simulink model "MotorTestHarness"  (R2024b)
settings: Solver=VariableStepAuto  StartTime=0.0  StopTime=300  RelTol=1e-3  AbsTol=1e-3
libraries: fl_lib x12, nesl_utility x6, simulink x2
settings Model: Creator=saprasad  LastModifiedBy=jjha
settings SolverCC: AutoScaleAbsTol=off  AlgebraicLoopSolver=TrustRegion  MaxZcPerStep=1
settings DebuggingCC: UnconnectedInputMsg=warning  UnconnectedOutputMsg=warning  UnconnectedLineMsg=warning  SymbolicDimsDataTypeCodeGenerationDiagnostic=none
settings ModelReferenceCC: EnableRefExpFcnMdlSchedulingChecks=on
settings SFSimCC: CustomCodeUndefinedFunction=UseInterfaceOnly
settings RTWCC: GPUComputeCapability=3.5  DLArmComputeVersion=19.05
settings SimscapeCC: SimscapeLogType=all  SimscapeLogSimulationStatistics=on  SimscapeLogDataHistory=10000

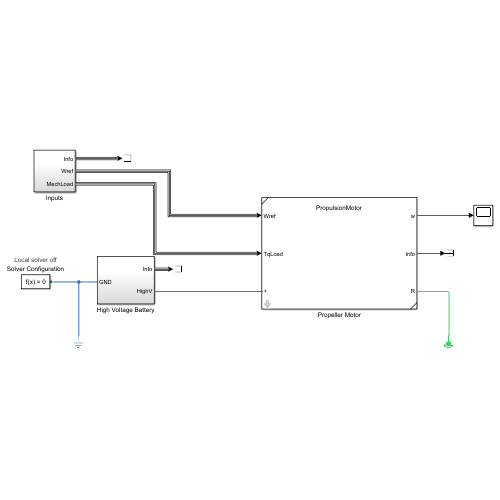
[thumbnail: Simulink's stored preview of the top-level diagram]
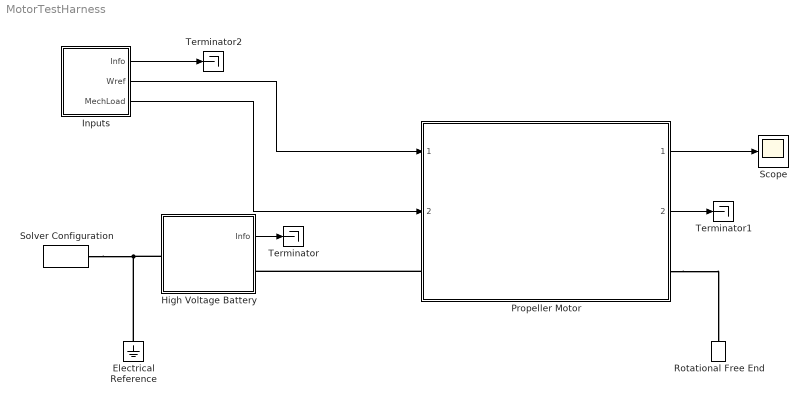
== system MotorTestHarness ==
  Electrical Reference : fl_lib/Electrical/Electrical Elements/Electrical Reference
  High Voltage Battery : Subsystem
  Inputs : Subsystem
  Propeller Motor : Subsystem  ReferencedSubsystem=PropulsionMotor  Kp=0.0129  Ki=0.00568  Kd=0.00644  N=382
  Rotational Free End : fl_lib/Mechanical/Rotational Elements/Rotational Free End  w_specify=off  w_priority=None  w=0 rad/s  w_nominal_specify=off  w_nominal_value=1  w_nominal_unit=rad/s
  Scope : Scope
  Solver Configuration : nesl_utility/Solver Configuration  PhysicalDomain=network_engine_domain  SubClassName=solver  LeftPortType=input  RightPortType=generic  Tones=[]  Harmonics=[]  SimulateNoise=off  Profile=off  UseLocalSampling=off  EnableSwitchedLinearOptims=on  FrequencyDomain=off  UseCCode=off  RelTol=0.001  AbsTol=1e-06  MinStep=1e-09  ToWorkspace=off  RevertToSquareIcSolve=off  NumHomotopyIterations=100  PhasorMode=off  PhasorModeNumHarmonics=1  ConsistencySolver=NEWTON_XTOL_AFTER_FTOL  IndexReductionMethod=DerivativeReplacement  DoDC=off  ResidualTolerance=1e-09  ConsistencyTolSource=GLOBAL  ConsistencyAbsTol=0.001  ConsistencyRelTol=0.001  ConsistencyTolFactor=0.001  UseLocalSolver=off  LocalSolverChoice=NE_BACKWARD_EULER_ADVANCER  ResolveIndetEquations=on  FunctionEvalNumThread=1  LocalSolverSampleTime=0.001  DoFixedCost=off  MaxNonlinIter=3  MaxModeIter=2  ComputeImpulses=off  ImpulseIterations=2  LinearAlgebra=auto  LinearAlgebraNumThread=0  EquationFormulation=NE_TIME_EF  DelaysMemoryBudget=1024  AutomaticFiltering=on  FilteringTimeConstant=0.001  PartitionStorageMethod=AS_NEEDED  PartitionMemoryBudget=1024  PartitionMethod=ROBUST  MultibodyUseLocalSolver=off  MultibodyLocalSolverChoice=ODE1  MultibodyLocalSolverSampleTime=0.001
      settings: AttributesFormatString=Local solver %<UseLocalSolver>
  Terminator : Terminator
  Terminator1 : Terminator
  Terminator2 : Terminator
  wires:
  Inputs/2(Wref) -> Propeller Motor/1
  Inputs/1(Info) -> Terminator2/1
  Inputs/3(MechLoad) -> Propeller Motor/2
  High Voltage Battery/1(Info) -> Terminator/1
  Propeller Motor/1 -> Scope/1
  Propeller Motor/2 -> Terminator1/1
  connections:
  High Voltage Battery/LConn1 -- Electrical Reference/LConn1 -- Solver Configuration/RConn1
  Propeller Motor/LConn1 -- High Voltage Battery/RConn1
  Propeller Motor/RConn1 -- Rotational Free End/LConn1

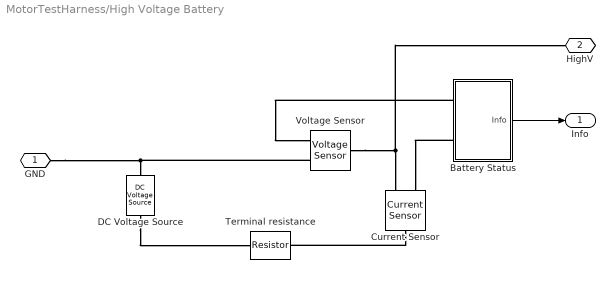
== system MotorTestHarness/High Voltage Battery ==
  Battery Status : Subsystem
  Current Sensor : fl_lib/Electrical/Electrical Sensors/Current Sensor
  DC Voltage Source : fl_lib/Electrical/Electrical Sources/DC Voltage Source  v0=420 V
      settings: AttributesFormatString=%<v0> [%<v0_unit>]
  Terminal resistance : fl_lib/Electrical/Electrical Elements/Resistor  R=0.01 Ohm  i_specify=off  i_priority=High  i=0 A  i_nominal_specify=off  i_nominal_value=1  i_nominal_unit=A  v_specify=off  v_priority=High  v=0 V  v_nominal_specify=off  v_nominal_value=1  v_nominal_unit=V
      settings: AttributesFormatString=%<R> [%<R_unit>]
  Voltage Sensor : fl_lib/Electrical/Electrical Sensors/Voltage Sensor
  GND : PMIOPort  Side=Left
  HighV : PMIOPort  Port=2  Side=Right
  Info : Outport
  wires:
  Battery Status/1(Info) -> Info/1
  connections:
  DC Voltage Source/RConn1 -- GND/RConn1 -- Voltage Sensor/RConn2
  Battery Status/LConn2 -- Current Sensor/RConn1
  Voltage Sensor/LConn1 -- HighV/RConn1 -- Current Sensor/RConn2
  Current Sensor/LConn1 -- Terminal resistance/RConn1
  DC Voltage Source/LConn1 -- Terminal resistance/LConn1
  Battery Status/LConn1 -- Voltage Sensor/RConn1

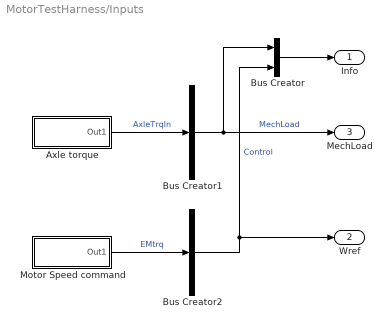
== system MotorTestHarness/Inputs ==
  Axle torque : Subsystem  mask(Continuous Multi-Step Signal){dataPoints=[0 20 0.1;60 100 0.25;105 200 0.15;205 300 0], deltaT=0.1}
      mask prompts: dataPoints "Data points"; deltaT "Interpolation step [s]"
      mask help:
      | This block generates a signal consisting of smoothly connected flat segments. Data points parameter takes an N-by-3 matrix where each row specifies a flat segment. First column and second column define start and end time of the segment, respectively. Third column defines the value of the segment. Second column can also be NaN to define a point value. Flat segments and point values are smoothly interpolated by Akima spline with the specified interpolation step.
      |
      | For example, a matrix [0 1 5; 3 nan 9; 6 8 7] for Data points defines a signal as follows. First row defines a flat segment from t=0 to t=1 of value 5. Second row defines a point at t=3 of value 9. Third row defines a flat segment from t=6 to t=8 of value 7.
      mask init:
      | sig = SignalDesigner("ContinuousMultiStep");
      | 
      | % Initialization function can access parameter names directly
      | sig.XYData = dataPoints;
      | sig.DeltaX = deltaT;
      | 
      | update(sig)
      | 
      | SignalSourceBlockCallback.setDataToLookupTableBlock( ...
      |   SignalObject = sig, ...
      |   PathToBlock = [gcb '/1-D Lookup Table']);
      mask DialogControl Control3 Prompt: horizontal spacer 1
      mask DialogControl Control4 Prompt: horizontal spacer 2
      mask DialogControl Control5 Prompt: horizontal spacer 3
      mask DialogControl PlotButton Prompt: Plot
      mask DialogControl PlotButton Callback: SignalSourceBlockCallback.plotContinuousMultiStep(gcb);
      mask Display: disp("Continuous" + newline + "Multi-Step")
  Bus Creator : BusCreator  Inputs=2
  Bus Creator1 : BusCreator  Inputs=1
  Bus Creator2 : BusCreator  Inputs=1
  Motor Speed command : Subsystem  mask(Continuous Multi-Step Signal){dataPoints=[0 20 0;60 100 100;105 200 50;205 300 0], deltaT=0.5}
      mask prompts: dataPoints "Data points"; deltaT "Interpolation step [s]"
      mask help:
      | This block generates a signal consisting of smoothly connected flat segments. Data points parameter takes an N-by-3 matrix where each row specifies a flat segment. First column and second column define start and end time of the segment, respectively. Third column defines the value of the segment. Second column can also be NaN to define a point value. Flat segments and point values are smoothly interpolated by Akima spline with the specified interpolation step.
      |
      | For example, a matrix [0 1 5; 3 nan 9; 6 8 7] for Data points defines a signal as follows. First row defines a flat segment from t=0 to t=1 of value 5. Second row defines a point at t=3 of value 9. Third row defines a flat segment from t=6 to t=8 of value 7.
      mask init: same as MotorTestHarness/Inputs/Axle torque
      mask DialogControl Control3 Prompt: horizontal spacer 1
      mask DialogControl Control4 Prompt: horizontal spacer 2
      mask DialogControl Control5 Prompt: horizontal spacer 3
      mask DialogControl PlotButton Prompt: Plot
      mask DialogControl PlotButton Callback: SignalSourceBlockCallback.plotContinuousMultiStep(gcb);
      mask Display: disp("Continuous" + newline + "Multi-Step")
  Info : Outport
  Wref : Outport  Port=2
  MechLoad : Outport  Port=3
  wires:
  Bus Creator/1 -> Info/1
  Motor Speed command/1(Out1) -> Bus Creator2/1  "EMtrq"
  Axle torque/1(Out1) -> Bus Creator1/1  "AxleTrqIn"
  Bus Creator1/1 -> Bus Creator/1, MechLoad/1  "MechLoad"
  Bus Creator2/1 -> Bus Creator/2, Wref/1  "Control"

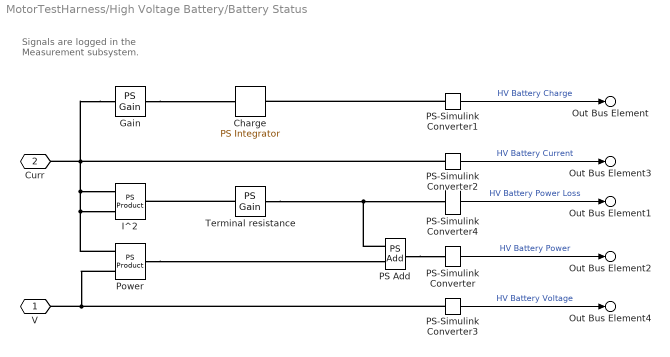
== system MotorTestHarness/High Voltage Battery/Battery Status ==
  note: Signals are logged in
      | the Measurement subsystem.
  Charge : fl_lib/Physical Signals/Linear Operators/PS Integrator  reset_method=foundation.enum.IntegratorResetSpec.None  initial_condition_spec=foundation.enum.IntegratorICSpec.Internal  saturation_spec=foundation.enum.IntegratorSaturationSpec.None  saturation_source_spec=foundation.enum.IntegratorSaturationSourceSpec.Internal  x0=0 A*hr  xu=inf s  xl=-inf s
      settings: AttributesFormatString=%<x0> [%<x0_unit>]
  Gain : fl_lib/Physical Signals/Functions/PS Gain  gain=-1
      settings: AttributesFormatString=%<gain>
  I^2 : fl_lib/Physical Signals/Functions/PS Product
  PS Add : fl_lib/Physical Signals/Functions/PS Add
  PS-Simulink Converter : nesl_utility/PS-Simulink Converter  PhysicalDomain=network_engine_domain  SubClassName=ps_output  LeftPortType=input  RightPortType=output  PseudoPeriodic=off  Frequencies=[]  VectorFormat=1-D array  Unit=kW  AffineConversion=off
  PS-Simulink Converter1 : nesl_utility/PS-Simulink Converter  PhysicalDomain=network_engine_domain  SubClassName=ps_output  LeftPortType=input  RightPortType=output  PseudoPeriodic=off  Frequencies=[]  VectorFormat=1-D array  Unit=A*hr  AffineConversion=off
  PS-Simulink Converter2 : nesl_utility/PS-Simulink Converter  PhysicalDomain=network_engine_domain  SubClassName=ps_output  LeftPortType=input  RightPortType=output  PseudoPeriodic=off  Frequencies=[]  VectorFormat=1-D array  Unit=A  AffineConversion=off
  PS-Simulink Converter3 : nesl_utility/PS-Simulink Converter  PhysicalDomain=network_engine_domain  SubClassName=ps_output  LeftPortType=input  RightPortType=output  PseudoPeriodic=off  Frequencies=[]  VectorFormat=1-D array  Unit=V  AffineConversion=off
  PS-Simulink Converter4 : nesl_utility/PS-Simulink Converter  PhysicalDomain=network_engine_domain  SubClassName=ps_output  LeftPortType=input  RightPortType=output  PseudoPeriodic=off  Frequencies=[]  VectorFormat=1-D array  Unit=W  AffineConversion=off
  Power : fl_lib/Physical Signals/Functions/PS Product
  Terminal resistance : fl_lib/Physical Signals/Functions/PS Gain  gain=0.01 Ohm
      settings: AttributesFormatString=%<gain> [%<gain_unit>]
  V : PMIOPort  Side=Left
  Curr : PMIOPort  Port=2  Side=Left
  Out Bus Element : Outport  PortName=Info  Element=Charge
      settings: AttributesFormatString=%<Unit>
  Out Bus Element3 : Outport  PortName=Info  Element=Current
      settings: AttributesFormatString=%<Unit>
  Out Bus Element1 : Outport  PortName=Info  Element=PowerLoss
      settings: AttributesFormatString=%<Unit>
  Out Bus Element2 : Outport  PortName=Info  Element=Power
      settings: AttributesFormatString=%<Unit>
  Out Bus Element4 : Outport  PortName=Info  Element=Voltage
      settings: AttributesFormatString=%<Unit>
  wires:
  PS-Simulink Converter3/1 -> Out Bus Element4/1  "HV Battery Voltage"
  PS-Simulink Converter2/1 -> Out Bus Element3/1  "HV Battery Current"
  PS-Simulink Converter4/1 -> Out Bus Element1/1  "HV Battery Power Loss"
  PS-Simulink Converter1/1 -> Out Bus Element/1  "HV Battery Charge"
  PS-Simulink Converter/1 -> Out Bus Element2/1  "HV Battery Power"
  connections:
  Power/RConn1 -- PS Add/LConn2
  PS Add/RConn1 -- PS-Simulink Converter/LConn1
  Terminal resistance/LConn1 -- I^2/RConn1
  PS-Simulink Converter1/LConn1 -- Charge/RConn1
  Gain/RConn1 -- Charge/LConn1
  PS Add/LConn1 -- Terminal resistance/RConn1 -- PS-Simulink Converter4/LConn1
  Power/LConn1 -- V/RConn1 -- PS-Simulink Converter3/LConn1
  Gain/LConn1 -- PS-Simulink Converter2/LConn1 -- Curr/RConn1 -- I^2/LConn1 -- Power/LConn2 -- I^2/LConn2

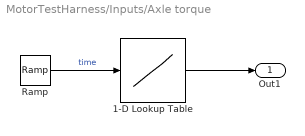
== system MotorTestHarness/Inputs/Axle torque ==
  1-D Lookup Table : Lookup_n-D  NumberOfTableDimensions=1  BreakpointsForDimension1="[0            20          20.1          20.2          20.3          20.4          20.5          20.6          20.7          20.8          20.9            21          21.1          21.2          21.3          21.4          21.5          21.6          21.7          21.8          21.9            22          22.1          22.2          22.3          22.4          22.5          22.6          22.7          22.8          22.9            23          23.1          23.2          23.3          23.4          23.5          23.6          23.7          23.8          23.9            24          24.1          24.2          24.3          24.4          24.5          24.6          24.7          24.8          24.9            25          25.1          25.2          25.3          25.4          25.5          25.6          25.7          25.8          25.9            26          26.1          26.2          26.3          26.4          26.5          26.6          26.7          26.8          26.9            27          27.1          27.2          27.3          27.4          27.5          27.6          27.7          27.8          27.9            28          28.1          28.2          28.3          28.4          28.5          28.6          28.7          28.8          28.9            29          29.1          29.2          29.3          29.4          29.5          29.6          29.7          29.8          29.9            30          30.1          30.2          30.3          30.4          30.5          30.6          30.7          30.8          30.9            31          31.1          31.2          31.3          31.4          31.5          31.6          31.7          31.8          31.9            32          32.1          32.2          32.3          32.4          32.5          32.6          32.7          32.8          32.9            33          33.1          33.2          33.3          33.4          33.5          33.6          33.7          33.8          33.9            34          34.1          34.2          34.3          34.4          34.5          34.6          34.7          34.8          34.9            35          35.1          35.2          35.3          35.4          35.5          35.6          35.7          35.8          35.9            36          36.1          36.2          36.3          36.4          36.5          36.6          36.7          36.8          36.9            37          37.1          37.2          37.3          37.4          37.5          37.6          37.7          37.8          37.9            38          38.1          38.2          38.3          38.4          38.5          38.6          38.7          38.8          38.9            39          39.1          39.2          39.3          39.4          39.5          39.6          39.7          39.8          39.9            40          40.1          40.2          40.3          40.4          40.5          40.6          40.7          40.8          40.9            41          41.1          41.2          41.3          41.4          41.5          41.6          41.7          41.8          41.9            42          42.1          42.2          42.3          42.4          42.5          42.6          42.7          42.8          42.9            43          43.1          43.2          43.3          43.4          43.5          43.6          43.7          43.8          43.9            44          44.1          44.2          44.3          44.4          44.5          44.6          44.7          44.8          44.9            45          45.1          45.2          45.3          45.4          45.5          45.6          45.7          45.8          45.9            46          46.1          46.2          46.3          46.4          46.5          46.6          46.7          46.8          46.9            47          47.1          47.2          47.3          47.4          47.5          47.6          47.7          47.8          47.9            48          48.1          48.2          48.3          48.4 ...(+3059 chars)]"  Table="[0.1         0.1         0.1     0.10001     0.10003     0.10004     0.10007      0.1001     0.10014     0.10018     0.10022     0.10028     0.10033      0.1004     0.10047     0.10054     0.10062      0.1007     0.10079     0.10088     0.10098     0.10109      0.1012     0.10131     0.10143     0.10156     0.10168     0.10182     0.10196      0.1021     0.10225      0.1024     0.10256     0.10273     0.10289     0.10307     0.10324     0.10343     0.10361      0.1038       0.104      0.1042      0.1044     0.10461     0.10483     0.10505     0.10527     0.10549     0.10573     0.10596      0.1062     0.10645     0.10669     0.10695      0.1072     0.10746     0.10773       0.108     0.10827     0.10855     0.10883     0.10911      0.1094     0.10969     0.10999     0.11029      0.1106      0.1109     0.11122     0.11153     0.11185     0.11217      0.1125     0.11283     0.11316      0.1135     0.11384     0.11419     0.11454     0.11489     0.11524      0.1156     0.11596     0.11633      0.1167     0.11707     0.11744     0.11782      0.1182     0.11859     0.11897     0.11936     0.11976     0.12015     0.12055     0.12096     0.12136     0.12177     0.12218      0.1226     0.12302     0.12344     0.12386     0.12429     0.12472     0.12515     0.12558     0.12602     0.12646      0.1269     0.12734     0.12779     0.12824     0.12869     0.12915     0.12961     0.13007     0.13053     0.13099     0.13146     0.13193      0.1324     0.13287     0.13335     0.13383     0.13431     0.13479     0.13527     0.13576     0.13625     0.13674     0.13723     0.13773     0.13822     0.13872     0.13922     0.13972     0.14023     0.14073     0.14124     0.14175     0.14226     0.14278     0.14329     0.14381     0.14432     0.14484     0.14536     0.14589     0.14641     0.14693     0.14746     0.14799     0.14852     0.14905     0.14958     0.15011     0.15065     0.15119     0.15172     0.15226      0.1528     0.15334     0.15388     0.15442     0.15497     0.15551     0.15606     0.15661     0.15715      0.1577     0.15825      0.1588     0.15935      0.1599     0.16046     0.16101     0.16156     0.16212     0.16267     0.16323     0.16379     0.16434      0.1649     0.16546     0.16602     0.16658     0.16714      0.1677     0.16826     0.16882     0.16938     0.16994      0.1705     0.17106     0.17163     0.17219     0.17275     0.17331     0.17388     0.17444       0.175     0.17556     0.17612     0.17669     0.17725     0.17781     0.17837     0.17894      0.1795     0.18006     0.18062     0.18118     0.18174      0.1823     0.18286     0.18342     0.18398     0.18454      0.1851     0.18566     0.18621     0.18677     0.18733     0.18788     0.18844     0.18899     0.18954      0.1901     0.19065      0.1912     0.19175      0.1923     0.19285     0.19339     0.19394     0.19449     0.19503     0.19558     0.19612     0.19666      0.1972     0.19774     0.19828     0.19881     0.19935     0.19989     0.20042     0.20095     0.20148     0.20201     0.20254     0.20307     0.20359     0.20411     0.20464     0.20516     0.20568     0.20619     0.20671     0.20722     0.20774     0.20825     0.20876     0.20927     0.20977     0.21028     0.21078     0.21128     0.21178     0.21227     0.21277     0.21326     0.21375     0.21424     0.21473     0.21521     0.21569     0.21617     0.21665     0.21713      0.2176     0.21807     0.21854     0.21901     0.21947     0.21993     0.22039     0.22085     0.22131     0.22176     0.22221     0.22266      0.2231     0.22354     0.22398     0.22442     0.22485     0.22528     0.22571     0.22614     0.22656     0.22698      0.2274     0.22782     0.22823     0.22864     0.22904     0.22945     0.22985     0.23024     0.23064     0.23103     0.23141      0.2318     0.23218     0.23256     0.23293      0.2333     0.23367     0.23404      0.2344     0.23476     0.23511     0.23546     0.23581     0.23616      0.2365     0.23684     0.23717      0.2375     0.23783     0.23815 ...(+2060 chars)]"  InternalRulePriority=Speed  RndMeth=Simplest
  Ramp : simulink/Sources/Ramp  slope=1  start=0  InitialOutput=0
      settings: AttributesFormatString=|
      | Slope: %<slope>
      | Start time: %<start>
      | Initial output: %<InitialOutput>
  Out1 : Outport
  wires:
  Ramp/1 -> 1-D Lookup Table/1  "time"
  1-D Lookup Table/1 -> Out1/1

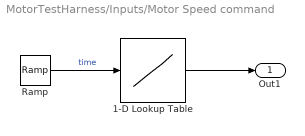
== system MotorTestHarness/Inputs/Motor Speed command ==
  1-D Lookup Table : Lookup_n-D  NumberOfTableDimensions=1  BreakpointsForDimension1="[0            20          20.5            21          21.5            22          22.5            23          23.5            24          24.5            25          25.5            26          26.5            27          27.5            28          28.5            29          29.5            30          30.5            31          31.5            32          32.5            33          33.5            34          34.5            35          35.5            36          36.5            37          37.5            38          38.5            39          39.5            40          40.5            41          41.5            42          42.5            43          43.5            44          44.5            45          45.5            46          46.5            47          47.5            48          48.5            49          49.5            50          50.5            51          51.5            52          52.5            53          53.5            54          54.5            55          55.5            56          56.5            57          57.5            58          58.5            59          59.5            60           100         100.5           101         101.5           102         102.5           103         103.5           104         104.5           105           200         200.5           201         201.5           202         202.5           203         203.5           204         204.5           205           300]"  Table="[0             0    0.04648438      0.184375     0.4113281         0.725      1.123047      1.603125      2.162891           2.8      3.512109      4.296875      5.151953         6.075      7.063672      8.115625      9.228516          10.4      11.62773      12.90938      14.24258        15.625       17.0543      18.52813      20.04414          21.6      23.19336      24.82187       26.4832        28.175      29.89492      31.64062      33.40977          35.2      37.00898      38.83437      40.67383        42.525      44.38555      46.25313      48.12539            50      51.87461      53.74687      55.61445        57.475      59.32617      61.16562      62.99102          64.8      66.59023      68.35938      70.10508        71.825       73.5168      75.17813      76.80664          78.4      79.95586      81.47188       82.9457        84.375      85.75742      87.09063      88.37227          89.6      90.77148      91.88437      92.93633        93.925      94.84805      95.70312      96.48789          97.2      97.83711      98.39688      98.87695        99.275      99.58867      99.81562      99.95352           100           100          98.6          94.8          89.2          82.4            75          67.6          60.8          55.2          51.4            50            50          48.6          44.8          39.2          32.4            25          17.6          10.8           5.2           1.4             0             0]"  InternalRulePriority=Speed  RndMeth=Simplest
  Ramp : simulink/Sources/Ramp  slope=1  start=0  InitialOutput=0
      settings: AttributesFormatString=|
      | Slope: %<slope>
      | Start time: %<start>
      | Initial output: %<InitialOutput>
  Out1 : Outport
  wires:
  1-D Lookup Table/1 -> Out1/1
  Ramp/1 -> 1-D Lookup Table/1  "time"
